simulink model "R_SIPsim2021a"  (R2021a)
settings: Solver=VariableStepAuto  StartTime=0.0  StopTime=10.0  RelTol=1e-3
values from neighbouring files (symbols this model uses):
  soft_dynamics =     [dynamics_handle.mat]
settings Model: Creator=Utente  LastModifiedBy=Utente

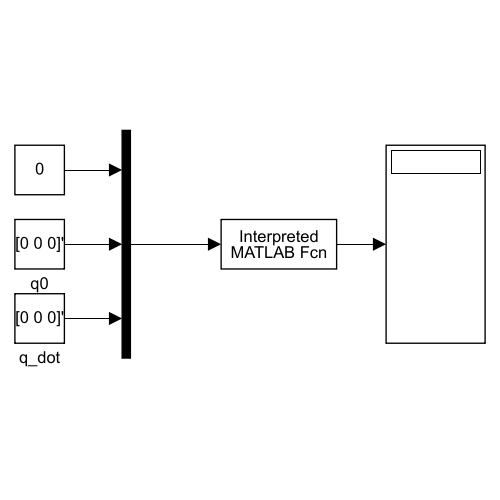
[thumbnail: Simulink's stored preview of the top-level diagram]
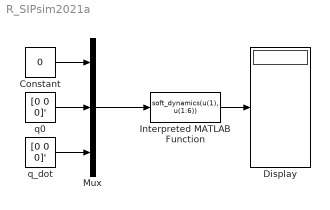
== system R_SIPsim2021a ==
  Constant : Constant  Value=0
  Display : Display
  Interpreted MATLAB Function : MATLABFcn  MATLABFcn=soft_dynamics(u(1), u(1:6))
  Mux : Mux  Inputs=3
  q0 : Constant  Value=[0 0 0]'
  q_dot : Constant  Value=[0 0 0]'
  wires:
  q0/1 -> Mux/2
  q_dot/1 -> Mux/3
  Mux/1 -> Interpreted MATLAB Function/1
  Constant/1 -> Mux/1
  Interpreted MATLAB Function/1 -> Display/1
